simulink model "AdaptiveMPC_Model_Jan11"  (R2019a)
settings: Solver=VariableStepAuto  StartTime=0.0  StopTime=10.0  RelTol=1e-3
libraries: sailbot_library x19, mpclib x1
settings Model: Creator=ronak  LastModifiedBy=ronak

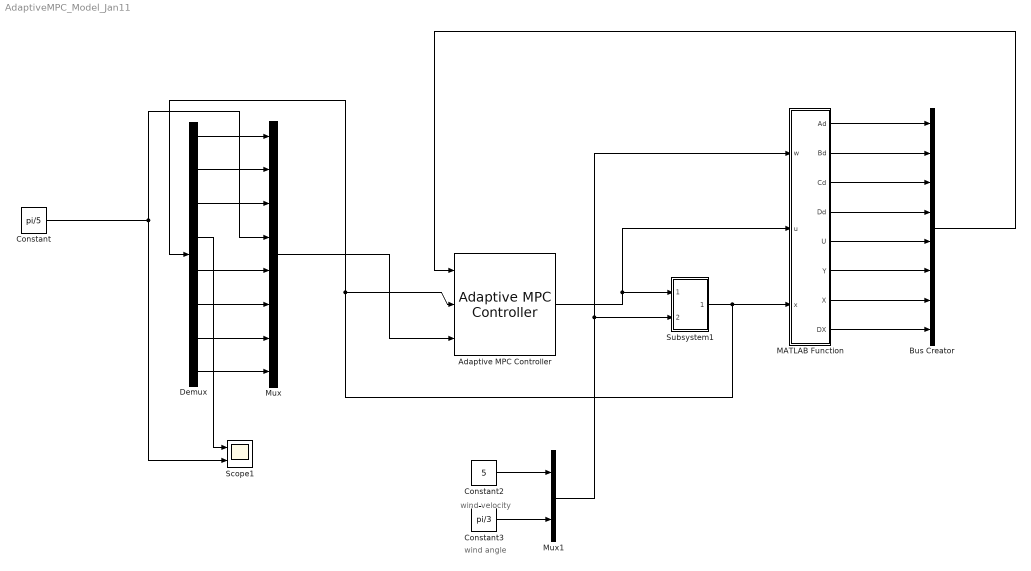
== system AdaptiveMPC_Model_Jan11 ==
  note: wind velocity
  note: wind angle
  Adaptive MPC Controller : mpclib/Adaptive MPC Controller  SCDEnableBlockLinearizationSpecification=on  mpcobj=mpc2  enable_value=0  updateMPCinCallerWorkspace=on  md_inport=off  mv_inport=off  uref_inport=off  return_cost=off  return_mvseq=off  return_qpstatus=off  return_xseq=off  return_state=off  return_ovseq=off  state_inport=off  isltv_plant=off  umin_inport=off  umax_inport=off  ymin_inport=off  ymax_inport=off  cc_inport=off  ywt_inport=off  uwt_inport=off  duwt_inport=off  rhoeps_inport=off  pm_inport=off  MaximumP=10  HorizonChoice=FixedHorizon  BlockDataType=double  SampleTimeInherited=off  switch_inport=off
      settings: SourceProductName=MATLAB Runtime - Model Predictive Control Toolbox Addin  SourceProductBaseCode=Missing
  Bus Creator : BusCreator  Inputs=8
  Constant : Constant  Value=pi/5
  Constant2 : Constant  Value=5
  Constant3 : Constant  Value=pi/3
  Demux : Demux  Outputs=8
  MATLAB Function : MATLAB Function  TreatAsAtomicUnit=on
  Mux : Mux  Inputs=8
  Mux1 : Mux  Inputs=2
  Scope1 : Scope  NumInputPorts=2
  Subsystem1 : Subsystem
  wires:
  Mux/1 -> Adaptive MPC Controller/3
  MATLAB Function/6(Y) -> Bus Creator/6
  MATLAB Function/8(DX) -> Bus Creator/8
  MATLAB Function/4(Dd) -> Bus Creator/4
  MATLAB Function/5(U) -> Bus Creator/5
  Bus Creator/1 -> Adaptive MPC Controller/1
  MATLAB Function/7(X) -> Bus Creator/7
  MATLAB Function/2(Bd) -> Bus Creator/2
  Constant2/1 -> Mux1/1
  Demux/1 -> Mux/1
  Demux/2 -> Mux/2
  Demux/7 -> Mux/7
  Demux/3 -> Mux/3
  Mux1/1 -> Subsystem1/2(In2), MATLAB Function/1(w)
  Adaptive MPC Controller/1 -> MATLAB Function/2(u), Subsystem1/1(In1)
  Demux/4 -> Scope1/1
  Demux/6 -> Mux/6
  Demux/8 -> Mux/8
  Demux/5 -> Mux/5
  Constant/1 -> Scope1/2, Mux/4
  Subsystem1/1(Out2) -> MATLAB Function/3(x), Adaptive MPC Controller/2, Demux/1
  Constant3/1 -> Mux1/2
  MATLAB Function/1(Ad) -> Bus Creator/1
  MATLAB Function/3(Cd) -> Bus Creator/3

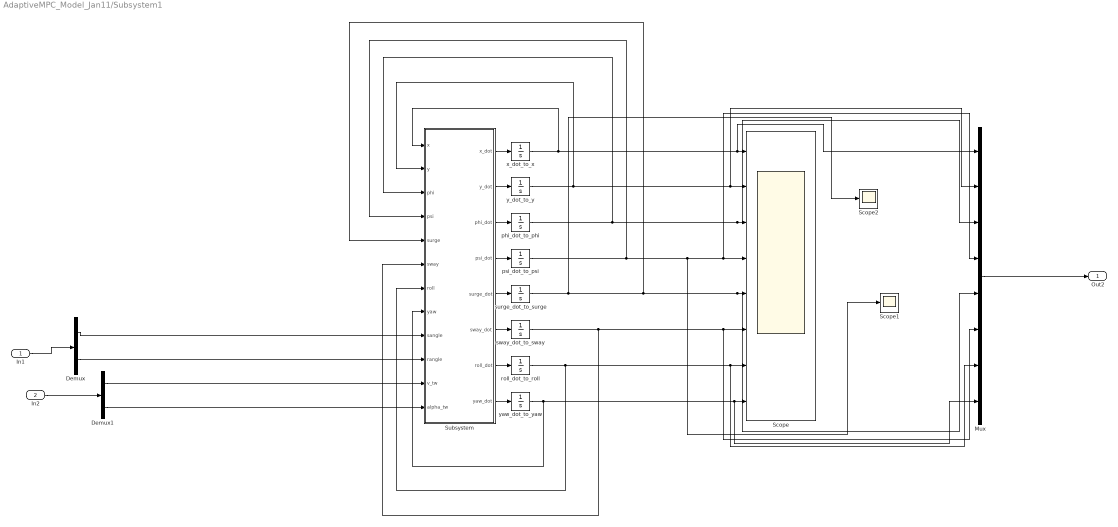
== system AdaptiveMPC_Model_Jan11/Subsystem1 ==
  In1 : Inport
  In2 : Inport  Port=2
  Demux : Demux  Outputs=2
  Demux1 : Demux  Outputs=2
  Mux : Mux  Inputs=8
  Scope : Scope  NumInputPorts=8
  Scope1 : Scope
  Scope2 : Scope
  Subsystem : Subsystem
  phi_dot_to_phi : Integrator
  psi_dot_to_psi : Integrator
  roll_dot_to_roll : Integrator
  surge_dot_to_surge : Integrator
  sway_dot_to_sway : Integrator
  x_dot_to_x : Integrator
  y_dot_to_y : Integrator
  yaw_dot_to_yaw : Integrator
  Out2 : Outport
  wires:
  x_dot_to_x/1 -> Mux/1, Scope/1, Subsystem/1(x)
  y_dot_to_y/1 -> Scope/2, Mux/2, Subsystem/2(y)
  phi_dot_to_phi/1 -> Subsystem/3(phi), Mux/3, Scope/3
  sway_dot_to_sway/1 -> Scope/6, Mux/6, Subsystem/6(sway)
  Subsystem/5(surge_dot) -> surge_dot_to_surge/1
  yaw_dot_to_yaw/1 -> Scope/8, Mux/8, Subsystem/8(yaw)
  roll_dot_to_roll/1 -> Scope/7, Mux/7, Subsystem/7(roll)
  psi_dot_to_psi/1 -> Subsystem/4(psi), Scope1/1, Scope/4, Mux/4
  Subsystem/1(x_dot) -> x_dot_to_x/1
  surge_dot_to_surge/1 -> Scope2/1, Subsystem/5(surge), Mux/5, Scope/5
  Subsystem/8(yaw_dot) -> yaw_dot_to_yaw/1
  Subsystem/4(psi_dot) -> psi_dot_to_psi/1
  Subsystem/3(phi_dot) -> phi_dot_to_phi/1
  Subsystem/6(sway_dot) -> sway_dot_to_sway/1
  Subsystem/2(y_dot) -> y_dot_to_y/1
  Subsystem/7(roll_dot) -> roll_dot_to_roll/1
  Mux/1 -> Out2/1
  Demux/1 -> Subsystem/9(sangle)
  Demux/2 -> Subsystem/10(rangle)
  In1/1 -> Demux/1
  Demux1/1 -> Subsystem/11(v_tw)
  Demux1/2 -> Subsystem/12(alpha_tw)
  In2/1 -> Demux1/1

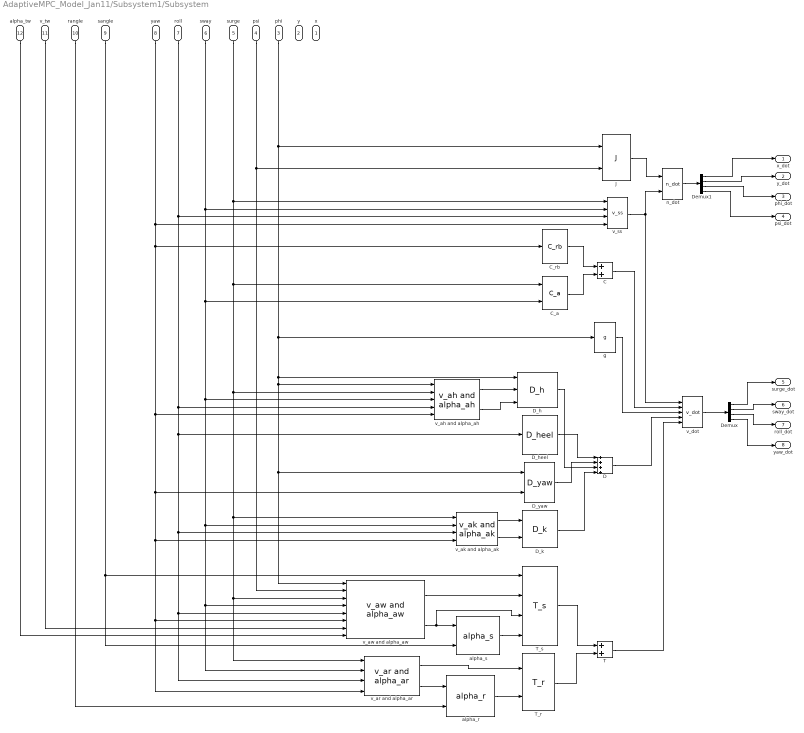
== system AdaptiveMPC_Model_Jan11/Subsystem1/Subsystem ==
  x : Inport
  y : Inport  Port=2
  phi : Inport  Port=3
  psi : Inport  Port=4
  surge : Inport  Port=5
  sway : Inport  Port=6
  roll : Inport  Port=7
  yaw : Inport  Port=8
  sangle : Inport  Port=9
  rangle : Inport  Port=10
  v_tw : Inport  Port=11
  alpha_tw : Inport  Port=12
  C : Sum
  C_a : sailbot_library/C_a  SystemSampleTime=-1
  C_rb : sailbot_library/C_rb  SystemSampleTime=-1
  D : Sum  Inputs=4
  D_h : sailbot_library/D_h  SystemSampleTime=-1
  "D_heel " : sailbot_library/D_heel   SystemSampleTime=-1
  D_k : sailbot_library/D_k  SystemSampleTime=-1
  D_yaw : sailbot_library/D_yaw  SystemSampleTime=-1
  Demux : Demux
  Demux1 : Demux
  J : sailbot_library/J  SystemSampleTime=-1
  T : Sum
  T_r : sailbot_library/T_r  SystemSampleTime=-1
  "T_s " : sailbot_library/T_s   SystemSampleTime=-1
  alpha_r : sailbot_library/alpha_r  SystemSampleTime=-1
  alpha_s : sailbot_library/alpha_s  SystemSampleTime=-1
  g : sailbot_library/g  SystemSampleTime=-1
  n_dot : sailbot_library/n_dot  SystemSampleTime=-1
  v_ah and alpha_ah : sailbot_library/v_ah and alpha_ah  SystemSampleTime=-1
  v_ak and alpha_ak : sailbot_library/v_ak and alpha_ak  SystemSampleTime=-1
  v_ar and alpha_ar : sailbot_library/v_ar and alpha_ar  SystemSampleTime=-1
  v_aw and alpha_aw : sailbot_library/v_aw and alpha_aw  SystemSampleTime=-1
  v_dot : sailbot_library/v_dot  SystemSampleTime=-1
  v_ss : sailbot_library/v_ss  SystemSampleTime=-1
  x_dot : Outport
  y_dot : Outport  Port=2
  phi_dot : Outport  Port=3
  psi_dot : Outport  Port=4
  surge_dot : Outport  Port=5
  sway_dot : Outport  Port=6
  roll_dot : Outport  Port=7
  yaw_dot : Outport  Port=8
  wires:
  alpha_s/1 -> "T_s "/4
  Demux/4 -> yaw_dot/1
  C/1 -> v_dot/2
  v_ah and alpha_ah/1 -> D_h/2
  D/1 -> v_dot/4
  v_aw and alpha_aw/1 -> "T_s "/2
  v_ak and alpha_ak/1 -> D_k/1
  v_ak and alpha_ak/2 -> D_k/2
  Demux/3 -> roll_dot/1
  C_a/1 -> C/2
  J/1 -> n_dot/1
  psi/1 -> v_aw and alpha_aw/2, J/2
  Demux1/4 -> psi_dot/1
  Demux1/2 -> y_dot/1
  T/1 -> v_dot/5
  v_aw and alpha_aw/2 -> "T_s "/3, alpha_s/1
  alpha_tw/1 -> v_aw and alpha_aw/8
  sway/1 -> v_ss/2, C_a/2, v_ah and alpha_ah/3, v_aw and alpha_aw/4, v_ar and alpha_ar/2, v_ak and alpha_ak/2
  alpha_r/1 -> T_r/2
  v_tw/1 -> v_aw and alpha_aw/7
  g/1 -> v_dot/3
  C_rb/1 -> C/1
  v_ah and alpha_ah/2 -> D_h/3
  v_ss/1 -> v_dot/1, n_dot/2
  n_dot/1 -> Demux1/1
  Demux1/3 -> phi_dot/1
  surge/1 -> v_ak and alpha_ak/1, v_aw and alpha_aw/3, v_ar and alpha_ar/1, v_ah and alpha_ah/2, C_a/1, v_ss/1
  Demux1/1 -> x_dot/1
  v_ar and alpha_ar/1 -> T_r/1
  rangle/1 -> alpha_r/2
  yaw/1 -> v_ss/4, D_yaw/2, v_ak and alpha_ak/4, v_ar and alpha_ar/4, v_aw and alpha_aw/6, v_ah and alpha_ah/5, C_rb/1
  phi/1 -> J/1, D_h/1, D_yaw/1, v_aw and alpha_aw/1, v_ah and alpha_ah/1, g/1
  Demux/1 -> surge_dot/1
  sangle/1 -> "T_s "/1, alpha_s/2
  v_ar and alpha_ar/2 -> alpha_r/1
  Demux/2 -> sway_dot/1
  roll/1 -> v_ss/3, v_ah and alpha_ah/4, "D_heel "/1, v_ak and alpha_ak/3, v_aw and alpha_aw/5, v_ar and alpha_ar/3
  v_dot/1 -> Demux/1
  "D_heel "/1 -> D/1
  D_yaw/1 -> D/2
  D_h/1 -> D/3
  D_k/1 -> D/4
  T_r/1 -> T/2
  "T_s "/1 -> T/1

== matlab function AdaptiveMPC_Model_Jan11/MATLAB Function ==
  data: w input; u input; Ad output; x input; Bd output; Cd output; Dd output; U output; Y output; X output; DX output
function [Ad,Bd,Cd,Dd,U,Y,X,DX] = Linearizer(w, u, x)

for i = 1:8
    if(x(i) == 0)
        x(i) = 0.01
    end
end

u1 = u(1);
u2 = u(2);
u3 = w(1);
u4 = w(2);
x1 = x(1);
x2 = x(2);
x3 = x(3);
x4 = x(4);
x5 = x(5);
x6 = x(6);
x7 = x(7);
x8 = x(8);

Ac = A(u1,u2,u3,u4,x3,x4,x5,x6,x7,x8);
Bc = B(u1,u2,u3,u4,x3,x4,x5,x6,x7,x8);
Ts = 1;
Cc = eye(8);
Dc = zeros(8,2);
% Generate discrete-time model
nx = size(Ac,1);
nu = size(Bc,2);
M = expm([[Ac Bc]*Ts; zeros(nu,nx+nu)]);
Ad = M(1:nx,1:nx);
Bd = M(1:nx,nx+1:nx+nu);
Cd = Cc;
Dd = Dc;
if(
% Nominal conditions for discrete-time plant
X = x;
U = u;
Y = Cd*x + Dd*u;
DX = Ad*x+Bd*u-x;
